simulink model "DIMR_ordinary"  (R2024b)
settings: Solver=daessc  StartTime=0.0  StopTime=20  RelTol=1e-3
values from neighbouring files (symbols this model uses):
  d_m0 = 0.12787808985686    (= 0.127878089857)    [DIMR_main.m]
  d_m_cmd = 0.12787808985686    (= 0.127878089857)    [DIMR_main.m]
  dis_cmd = 3    [DIMR_main.m]
  phi_cmd = 0*pi/180    (= 0)    [DIMR_main.m]
  theta_f0 = 0    [DIMR_main.m]
  theta_f_cmd = 0.037940459    [DIMR_main.m]
  theta_p0 = 0*pi/180    (= 0)    [DIMR_main.m]
  theta_p_cmd = -0.037940459    [DIMR_main.m]
undefined symbols (not defined in the file or in its folder): Ac, Dc, DiscIntNeverNeededParam, dspblkCoreblockFVToolHelper, g, g_ext, g_fork, g_lift, g_reac, g_spado, g_yaw, gcbh, K_fd, K_fp, K_md, K_mp, K_pd, K_pp, K_wd, K_wp, K_yd, K_yp, Kc, L_bx, L_by, L_bz, L_ex, L_ey, L_ez, L_fg, L_fh, L_fx, L_fy, L_fz, L_lx, L_ly, L_lz, L_mx, L_my, L_mz, L_wt, M_f, M_n11, M_n21, M_n22, M_n33, M_n44, Mc, N_f, N_w, omega_c, R_wi, R_wo, T_control, Torque_limit_f, Torque_limit_l, Torque_limit_w, W_w, X, Y ... (+1)
libraries: sm_lib x50, nesl_utility x12, simulink x9, slctrl_autotuning x1, slpidlib x1
(part 1 of 3)
settings Model: Creator=ITO  LastModifiedBy=Sergio Quintero
settings RTWCC: GPUComputeCapability=3.5

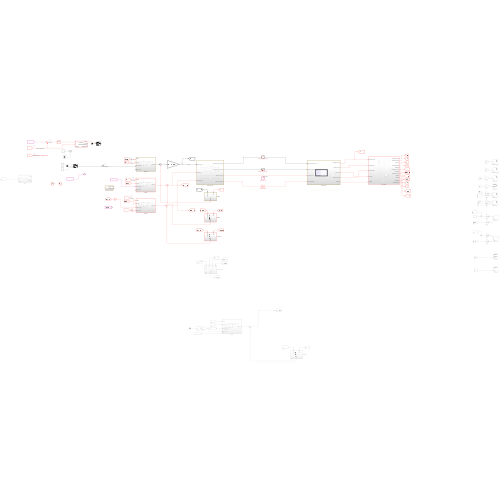
[thumbnail: Simulink's stored preview of the top-level diagram]
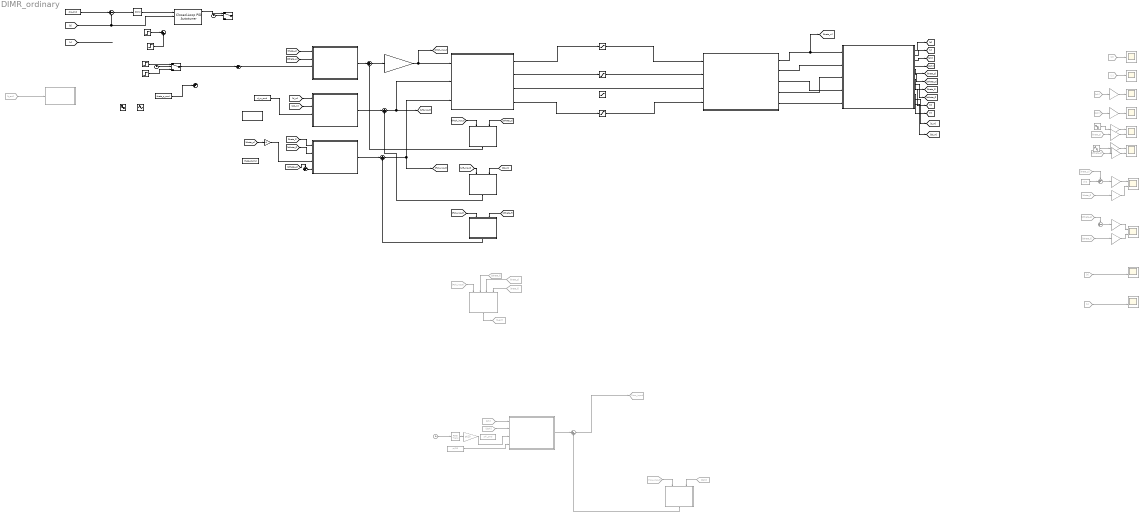
== system DIMR_ordinary ==
  Calc_states : Subsystem
  Clock : Clock  Commented=on
  Clock1 : Clock
  Clock2 : Clock
  Closed-Loop PID Autotuner : slctrl_autotuning/Closed-Loop PID Autotuner  PIDType=PD  PIDForm=Parallel  TimeDomain=discrete-time  DiscreteTs=T_control  TuningTs=0.2  UseTuningTs=off  IntegratorFormula=Forward Euler  FilterFormula=Forward Euler  ContinuousTs=0.02  Bandwidth=1  UseExternalWC=off  TargetPM=60  UseExternalPM=off  UseExternalAchievedPM=on  ExperimentMode=Superposition  PlantType=Stable  PlantSign=Positive  AmpSine=0.05  UseExternalAmpSine=off  UseExternalFRD=off  UseExternalU0=off  UseCompanion=off  NotDeployTuningModule=off  UsePLCCoder=off  OutputMode=control action + perturbation  BlockDataType=double  UseConnectedPID=on  blockpath=[]  tunedP=0  tunedI=0  tunedD=0  tunedN=100  tunedPM=0  EstimationWindowSize=3  UseExternalTuningParams=off  SingleMultiRateVariant=SingleSamplingRate  NumEstimationPeriods=4  NumSettlingPeriods=2  NumOfPRBSPeriod=1  PRBSSignalOrder=12  ExperimentModeVariant=VariantSuperimposed  OutputChoice=VariantCandD  ConvergenceCalcVariant=ConvSuperpositionPRBSVariant
      settings: LibrarySourceBlock=slctrlblks/Autotuning/Closed-Loop PID Autotuner
  Constant : Constant  Value=theta_p_cmd
  Constant1 : Constant  Commented=on  Value=phi_cmd
  Constant2 : Constant  Value=theta_f_cmd
  Constant3 : Constant  Commented=on  Value=pi/2
  Constant4 : Constant  Commented=on  Value=pi/20
  Constant5 : Constant  Value=d_m_cmd
  Constant6 : Constant  Value=dis_cmd
  Fork DOB : Subsystem
  Fork PD : Subsystem
  Fork position : Scope  Commented=on  NumInputPorts=2
  Fork velocity : Scope  Commented=on  NumInputPorts=2
  From1 : From  Commented=on  GotoTag=dphi
  From10 : From  Commented=on  GotoTag=Yaw_input
  From14 : From  Commented=on  GotoTag=d
  From15 : From  Commented=on  GotoTag=v
  From16 : From  Commented=on  GotoTag=phi
  From17 : From  Commented=on  GotoTag=dphi
  From18 : From  Commented=on  GotoTag=theta_p
  From19 : From  Commented=on  GotoTag=dtheta_p
  From20 : From  Commented=on  GotoTag=theta_f
  From21 : From  Commented=on  GotoTag=dtheta_f
  From22 : From  Commented=on  GotoTag=theta_p
  From23 : From  Commented=on  GotoTag=dtheta_p
  From24 : From  Commented=on  GotoTag=X
  From25 : From  Commented=on  GotoTag=Y
  From31 : From  Commented=on  GotoTag=dtheta_f
  From32 : From  Commented=on  GotoTag=Fork_input
  From33 : From  Commented=on  GotoTag=t_ext
  From34 : From  Commented=on  GotoTag=theta_p
  From35 : From  Commented=on  GotoTag=theta_f
  From5 : From  Commented=on  GotoTag=phi
  From6 : From  Commented=on  GotoTag=dphi
  Gain : Gain  Gain=-M_n11/(M_n21+M_n11)
  Gain{1..8,10..11} (10 alike) : Gain  Commented=on  Gain=180/pi
  Gain12 : Gain  Gain=-1
  Gain9 : Gain  Commented=on  Gain=pi/20
  Goto11 : Goto  Commented=on  GotoTag=Yaw_input
  Goto17 : Goto  Commented=on  GotoTag=t_ext
  Lift DOB : Subsystem
  Lift PD : Subsystem
  Lift movement profile : Subsystem
  PID Controller : slpidlib/PID Controller  Controller=PD  Form=Parallel  TimeDomain=Discrete-time  UseExternalTs=off  SampleTime=T_control  IntegratorMethod=Forward Euler  FilterMethod=Forward Euler  ControllerParametersSource=internal  P=K_wp  I=1  UseKiTs=off  D=K_wd  UseExternalDerivativeSource=off  N=100  UseFilter=off  TunerSelectOption=Transfer Function Based (PID Tuner App)  InitialConditionSource=internal  InitialConditionForIntegrator=0  InitialConditionForFilter=0  DifferentiatorICPrevScaledInput=0  ExternalReset=none  TrackingMode=off  Kt=1  LimitOutput=off  SatLimitsSource=internal  UpperSaturationLimit=inf  LowerSaturationLimit=-inf  LinearizeAsGain=on  AntiWindupMode=none  Kb=1  LimitIntegrator=off  UpperIntegratorSaturationLimit=inf  LowerIntegratorSaturationLimit=-inf  POutMin=[]  POutMax=[]  IOutMin=[]  IOutMax=[]  DOutMin=[]  DOutMax=[]  NOutMin=[]  NOutMax=[]  SumOutMin=[]  SumOutMax=[]  SaturationOutMin=[]  SaturationOutMax=[]  PParamMin=[]  PParamMax=[]  IParamMin=[]  IParamMax=[]  DParamMin=[]  DParamMax=[]  NParamMin=[]  NParamMax=[]  KbParamMin=[]  KbParamMax=[]  KtParamMin=[]  KtParamMax=[]  KbOutMin=[]  KbOutMax=[]  KtOutMin=[]  KtOutMax=[]  IntegratorOutMin=[]  IntegratorOutMax=[]  FilterOutMin=[]  FilterOutMax=[]  SumI1OutMin=[]  SumI1OutMax=[]  SumI2OutMin=[]  SumI2OutMax=[]  SumI3OutMin=[]  SumI3OutMax=[]  SumI4OutMin=[]  SumI4OutMax=[]  SumDOutMin=[]  SumDOutMax=[]  DifferentiatorOutMin=[]  DifferentiatorOutMax=[]  FilterDiffOutCoefMin=[]  FilterDiffOutCoefMax=[]  ReciprocalOutMin=[]  ReciprocalOutMax=[]  SumDenOutMin=[]  SumDenOutMax=[]  SumNumOutMin=[]  SumNumOutMax=[]  DivideOutMin=[]  DivideOutMax=[]  UdiffTsProdOutMin=[]  UdiffTsProdOutMax=[]  NTsProdOutMin=[]  NTsProdOutMax=[]  UintegralTsProdOutMin=[]  UintegralTsProdOutMax=[]  UngainTsProdOutMin=[]  UngainTsProdOutMax=[]  ClampingZeroOutDataTypeStr=Inherit: Inherit via back propagation  ClampingZeroOutMin=[]  ClampingZeroOutMax=[]  FilterDenConstantOutDataTypeStr=Inherit: Inherit via back propagation  FilterDenConstantOutMin=[]  FilterDenConstantOutMax=[]  PCopyOutDataTypeStr=Inherit: Inherit via back propagation  PCopyOutMin=[]  PCopyOutMax=[]  NCopyOutDataTypeStr=Inherit: Inherit via back propagation  NCopyOutMin=[]  NCopyOutMax=[]  IntegratorContinuousStateAttributes=''  IntegratorStateMustResolveToSignalObject=off  IntegratorRTWStateStorageClass=Auto  FilterContinuousStateAttributes=''  FilterStateMustResolveToSignalObject=off  FilterRTWStateStorageClass=Auto  ParallelPVariant=InternalParameters  IdealPVariant=Disabled  IVariant=Disabled  DVariant=InternalParameters  IntegratorVariant=Disabled  SatVariant=Disabled  AWVariant=Disabled  PCopyVariant=Disabled  TRVariant=Disabled  FdbkBlocksVariant=Forward  IdealPFdbkVariant=Disabled  SatFdbkVariant=Disabled  DerivativeFilterVariant=Differentiator  NVariant=Passthrough  NCopyVariant=Disabled_SignalSpec  FilterICVariant=InternalICsDifferentiator  IntegratorICVariant=Disabled  ExternalResetVariant=Disabled  TRSumVariant=Passthrough  SumFdbkVariant=Disabled  SumVariant=Sum_PD  TsampFilterVariant=InternalTs  TsampNgainVariant=Passthrough  TsampIntegralVariant=Disabled_SignalSpec  ExternalSaturationOutDataTypeStr=Inherit: Same as second input  DerivativeSourceVariant=ErrorSignal  PreIntVariant=InternalPreInt
  Pitch PD : Subsystem
  Pitch position : Scope  Commented=on  NumInputPorts=2
  Pitch velocity : Scope  Commented=on  NumInputPorts=2
  Plant model : Subsystem
  RCC : Subsystem  Commented=on
  Rate Transition : RateTransition  Commented=on  OutPortSampleTime=T_control
  Reaction DOB : Subsystem  Commented=on
  SPADO : Subsystem
  Sine Wave : Sin  Amplitude=10*pi/180  SampleTime=T_control
  Sine Wave1 : Sin  Amplitude=10*pi/180  Phase=pi/2  SampleTime=T_control
  Sine Wave2 : Sin  Commented=on  Amplitude=10*pi/180  SampleTime=T_control
  Sine Wave3 : Sin  Commented=on  Amplitude=10*pi/180  Phase=pi/2  SampleTime=T_control
  Step : Step  Time=10  SampleTime=0
  Step1 : Step  Time=20  After=-1  SampleTime=0
  Step2 : Step  Time=0  After=theta_p_cmd*3/2  SampleTime=0
  Step3 : Step  Time=0  After=theta_p_cmd/2  SampleTime=0
  Sum{,2,7,10} (4 alike) : Sum  Inputs=|++
  Sum1 : Sum  Commented=on  Inputs=|++
  Sum3 : Sum  Inputs=++|
  Sum4 : Sum  Inputs=-+|
  Sum5 : Sum  Commented=on  Inputs=-+|
  Sum6 : Sum  Commented=on  Inputs=-+|
  Sum8 : Sum  Inputs=++|
  Sum9 : Sum  Inputs=|+-
  Switch : Switch  Criteria=u2 > Threshold  Threshold=5  SaturateOnIntegerOverflow=off  InputSameDT=off
  Switch1 : Switch  Criteria=u2 > Threshold  Threshold=5  SaturateOnIntegerOverflow=off  InputSameDT=off
  Transform_input : Subsystem
  Translational position : Scope  Commented=on
  Translational velocity : Scope  Commented=on
  X position : Scope  Commented=on  NumInputPorts=2
  Y position : Scope  Commented=on  NumInputPorts=2
  Yaw DOB : Subsystem  Commented=on
  Yaw PD : Subsystem  Commented=on
  Yaw Position : Scope  Commented=on
  Yaw rate : Scope  Commented=on
  torque_limit_fork : Saturate  UpperLimit=Torque_limit_f  LowerLimit=-Torque_limit_f
  torque_limit_left_wheel : Saturate  UpperLimit=Torque_limit_w  LowerLimit=-Torque_limit_w
  torque_limit_lift : Saturate  UpperLimit=Torque_limit_l  LowerLimit=-Torque_limit_l
  torque_limit_right_wheel : Saturate  UpperLimit=Torque_limit_w  LowerLimit=-Torque_limit_w
  wires:
  Plant model/4(Pitch_Euler_Angle) -> Calc_states/3(Pitch euler angle)
  Plant model/3(Fork_Angle) -> Calc_states/4(Fork angle)
  torque_limit_left_wheel/1 -> Plant model/2(Left_wheel_motor_torque)
  Plant model/1(Right_Wheel_Angle) -> [theta_w], Calc_states/1(Right wheel angle)
  Transform_input/4(Fork_motor_torque_ref) -> torque_limit_fork/1
  torque_limit_right_wheel/1 -> Plant model/1(Right_wheel_motor_torque)
  torque_limit_fork/1 -> Plant model/4(Fork_motor_torque)
  Transform_input/1(Right_wheel_motor_torque_ref) -> torque_limit_right_wheel/1
  Transform_input/2(Left_wheel_motor_torque_ref) -> torque_limit_left_wheel/1
  Plant model/2(Left_Wheel_Angle) -> Calc_states/2(Left wheel angle)
  Gain/1 -> [Pitch_input], Transform_input/1(Pitch_torque_ref)  "Tp_ref"
  Pitch PD/1(Torque_ref) -> Sum/1
  Sum/1 -> Gain/1
  Yaw PD/1(Torque_ref) -> Sum1/1
  Sum1/1 -> Goto11/1
  Yaw DOB/1(Est_dis) -> Sum1/2
  Fork PD/1(Torque_ref) -> Sum2/1
  Sum2/1 -> [Fork_input], Transform_input/3(Fork_torque_ref)
  Calc_states/1(Translational position) -> [d]
  Calc_states/2(Translational velocity) -> [v]
  Calc_states/3(Yaw angle) -> [phi]
  Calc_states/4(Yaw angular velocity) -> [dphi]
  Calc_states/5(Pitch angle) -> [theta_p]
  Calc_states/6(Pitch angular velocity) -> [dtheta_p]
  Calc_states/7(Fork position) -> [theta_f]
  Calc_states/8(Fork angular velocity) -> [dtheta_f]
  Calc_states/9(X position) -> [X]
  Calc_states/10(Y position) -> [Y]
  [dtheta_p] -> SPADO/2(Velocity)
  From1/1 -> Yaw DOB/2(Velocity)
  [dtheta_f] -> Fork DOB/2(Velocity)
  [dtheta_p] -> Pitch PD/2(Velocity)  "Pitch ang vel"
  [theta_p] -> Pitch PD/1(Position)  "Pitch angle"
  From5/1 -> Yaw PD/1(Position)
  From6/1 -> Yaw PD/2(Velocity)
  [theta_f] -> Fork PD/1(Position)  "Fork angle"
  [dtheta_f] -> Fork PD/2(Velocity)
  [Pitch_input] -> SPADO/1(Input Torque)
  From10/1 -> Yaw DOB/1(Input Torque)
  [Fork_input] -> Fork DOB/1(Input Torque)
  Sum4/1 -> Fork PD/4(Velocity_cmd)
  [theta_p] -> Gain12/1
  [dtheta_p] -> Sum4/1
  From14/1 -> Translational position/1  "res"
  From15/1 -> Translational velocity/1  "res"
  From16/1 -> Gain1/1
  From17/1 -> Gain2/1
  From18/1 -> Gain3/1
  From19/1 -> Gain4/1
  From20/1 -> Gain6/1
  From21/1 -> Gain8/1
  Sum5/1 -> Gain5/1
  Sum6/1 -> Gain7/1
  From22/1 -> Sum5/1
  Constant3/1 -> Sum5/2
  From23/1 -> Sum6/1
  Gain1/1 -> Yaw Position/1  "res"
  Gain2/1 -> Yaw rate/1  "res"
  Gain3/1 -> Pitch position/2  "res"
  Gain4/1 -> Pitch velocity/2  "res"
  Gain5/1 -> Fork position/1  "cmd"
  Gain6/1 -> Fork position/2  "res"
  Gain7/1 -> Fork velocity/1  "cmd"
  Gain8/1 -> Fork velocity/2  "res"
  Fork DOB/1(Est_dis) -> Sum2/2
  From24/1 -> X position/2  "res"
  From25/1 -> Y position/2  "res"
  Clock/1 -> Rate Transition/1
  Gain9/1 -> Yaw PD/3(Position_cmd)
  Rate Transition/1 -> Gain9/1
  Constant4/1 -> Yaw PD/4(Velocity_cmd)
  Gain10/1 -> Pitch position/1  "res"
  Sine Wave2/1 -> Gain10/1
  Gain11/1 -> Pitch velocity/1  "res"
  Sine Wave3/1 -> Gain11/1
  Lift PD/1(Torque_ref) -> Sum7/1
  Lift DOB/1(Est_dis) -> Sum7/2
  Sum7/1 -> [Lift_input], Transform_input/2(Lift_force_ref)
  [Lift_input] -> Lift DOB/1(Input Torque)
  Plant model/5(Lift_height) -> Calc_states/5(Lift height)
  Calc_states/11(Lift position) -> [d_m]
  Calc_states/12(Lift linear velocity) -> [dd_m]
  [dd_m] -> Lift DOB/2(Velocity)
  [d_m] -> Lift PD/1(Position)  "Lift_height"
  [dd_m] -> Lift PD/2(Velocity)
  Transform_input/3(Lift_motor_torque_ref) -> Plant model/3(Lift_motor_torque)  "Control height"
  [d] -> Closed-Loop PID Autotuner/2, Sum9/2  "Horizontal displacement"
  From31/1 -> Reaction DOB/2(Velocity)
  From32/1 -> Reaction DOB/1(Input Torque)
  Reaction DOB/1(Est_dis) -> Goto17/1
  From33/1 -> RCC/1(t_ext)
  From34/1 -> Reaction DOB/3(Theta_p)
  From35/1 -> Reaction DOB/4(Theta_f)
  Sum9/1 -> PID Controller/1  "Pos_error"
  PID Controller/1 -> Closed-Loop PID Autotuner/1
  Step/1 -> Sum10/1
  Step1/1 -> Sum10/2
  Constant6/1 -> Sum9/1
  Constant/1 -> Sum8/2
  Gain12/1 -> Fork PD/3(Position_cmd)
  Clock1/1 -> Switch/2
  Clock2/1 -> Switch1/2
  SPADO/1(Est_dis) -> Sum/2
  Sum3/1 -> Pitch PD/3(Position_cmd)  "Total_pitch"
  Step2/1 -> Switch/1
  Step3/1 -> Switch/3
  [v] -> ?  "Horizontal velocity"
  Switch/1 -> Sum3/2
  Constant5/1 -> Lift PD/3(Position_cmd)
  Closed-Loop PID Autotuner/1 -> Switch1/1

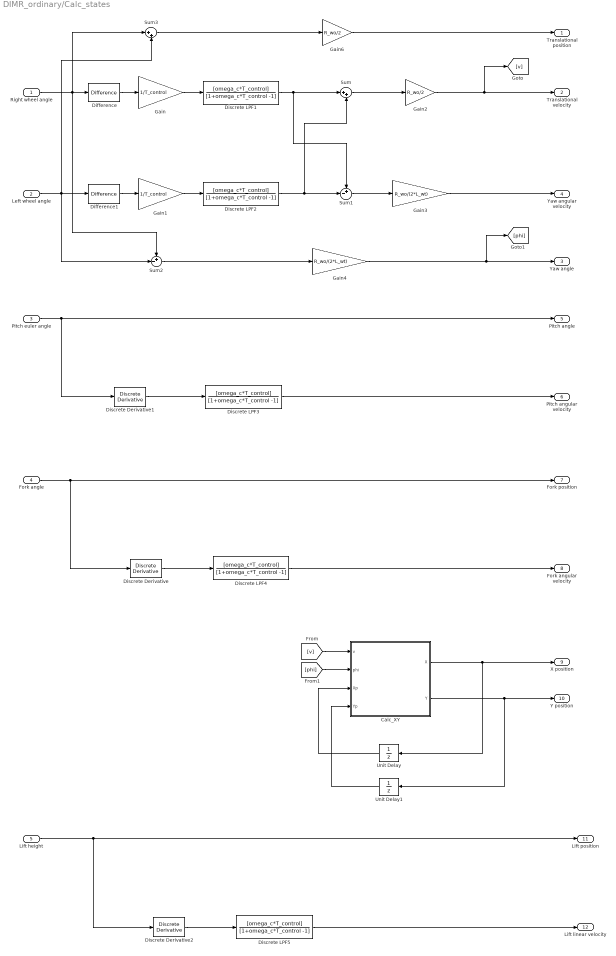
== system DIMR_ordinary/Calc_states ==
  Right wheel angle : Inport
  Left wheel angle : Inport  Port=2
  Pitch euler angle : Inport  Port=3
  Fork angle : Inport  Port=4
  Lift height : Inport  Port=5
  Calc_XY : MATLAB Function  TreatAsAtomicUnit=on
  Difference : simulink/Discrete/Difference  ICPrevInput=0.0  OutMin=[]  OutMax=[]  OutDataType=fixdt(1, 16)  OutScaling=2^-10  DoSatur=off
  Difference1 : simulink/Discrete/Difference  ICPrevInput=0.0  OutMin=[]  OutMax=[]  OutDataType=fixdt(1, 16)  OutScaling=2^-10  DoSatur=off
  Discrete Derivative : simulink/Discrete/Discrete Derivative  gainval=1.0  ICPrevScaledInput=theta_f0/T_control  OutMin=[]  OutMax=[]  OutDataType=fixdt(1, 16)  OutScaling=2^-10  DoSatur=off
  Discrete Derivative1 : simulink/Discrete/Discrete Derivative  gainval=1.0  ICPrevScaledInput=theta_p0/T_control  OutMin=[]  OutMax=[]  OutDataType=fixdt(1, 16)  OutScaling=2^-10  DoSatur=off
  Discrete Derivative2 : simulink/Discrete/Discrete Derivative  gainval=1.0  ICPrevScaledInput=d_m0/T_control  OutMin=[]  OutMax=[]  OutDataType=fixdt(1, 16)  OutScaling=2^-10  DoSatur=off
  Discrete LPF1 : DiscreteFilter  LoadFcn=dspblkCoreblockFVToolHelper(gcbh,'load');  Numerator=[omega_c*T_control]  Denominator=[1+omega_c*T_control -1]
      settings: CopyFcn=dspblkCoreblockFVToolHelper(gcbh,'copy');  DeleteFcn=dspblkCoreblockFVToolHelper(gcbh,'close');  ModelCloseFcn=dspblkCoreblockFVToolHelper(gcbh,'close');  PreSaveFcn=dspblkCoreblockFVToolHelper(gcbh,'presave');  PostSaveFcn=dspblkCoreblockFVToolHelper(gcbh,'postsave');  CloseFcn=dspblkCoreblockFVToolHelper(gcbh,'close');
  Discrete LPF2 : DiscreteFilter  Numerator=[omega_c*T_control]  Denominator=[1+omega_c*T_control -1]
  Discrete LPF3 : DiscreteFilter  Numerator=[omega_c*T_control]  Denominator=[1+omega_c*T_control -1]
  Discrete LPF4 : DiscreteFilter  Numerator=[omega_c*T_control]  Denominator=[1+omega_c*T_control -1]
  Discrete LPF5 : DiscreteFilter  LoadFcn=dspblkCoreblockFVToolHelper(gcbh,'load');  Numerator=[omega_c*T_control]  Denominator=[1+omega_c*T_control -1]
      settings: CopyFcn=dspblkCoreblockFVToolHelper(gcbh,'copy');  DeleteFcn=dspblkCoreblockFVToolHelper(gcbh,'close');  ModelCloseFcn=dspblkCoreblockFVToolHelper(gcbh,'close');  PreSaveFcn=dspblkCoreblockFVToolHelper(gcbh,'presave');  PostSaveFcn=dspblkCoreblockFVToolHelper(gcbh,'postsave');  CloseFcn=dspblkCoreblockFVToolHelper(gcbh,'close');
  Gain : Gain  Gain=1/T_control
  Gain1 : Gain  Gain=1/T_control
  Gain2 : Gain  Gain=R_wo/2
  Gain3 : Gain  Gain=R_wo/(2*L_wt)
  Gain4 : Gain  Gain=R_wo/(2*L_wt)
  Gain6 : Gain  Gain=R_wo/2
  Sum : Sum  Inputs=|++
  Sum1 : Sum  Inputs=+-|
  Sum2 : Sum  Inputs=+-|
  Sum3 : Sum  Inputs=|++
  Unit Delay : UnitDelay  SampleTime=T_control  HasFrameUpgradeWarning=on
  Unit Delay1 : UnitDelay  SampleTime=T_control  HasFrameUpgradeWarning=on
  Translational position : Outport
  Translational velocity : Outport  Port=2
  Yaw angle : Outport  Port=3
  Yaw angular velocity : Outport  Port=4
  Pitch angle : Outport  Port=5
  Pitch angular velocity : Outport  Port=6
  Fork position : Outport  Port=7
  Fork angular velocity : Outport  Port=8
  X position : Outport  Port=9
  Y position : Outport  Port=10
  Lift position : Outport  Port=11
  Lift linear velocity : Outport  Port=12
  wires:
  Right wheel angle/1 -> Sum3/1, Sum2/1, Difference/1
  Difference/1 -> Gain/1
  Gain/1 -> Discrete LPF1/1
  Difference1/1 -> Gain1/1
  Gain1/1 -> Discrete LPF2/1
  Left wheel angle/1 -> Sum3/2, Sum2/2, Difference1/1
  Discrete LPF1/1 -> Sum/1, Sum1/1
  Discrete LPF2/1 -> Sum1/2, Sum/2
  Sum/1 -> Gain2/1
  Gain2/1 -> Translational velocity/1, [v]
  Sum1/1 -> Gain3/1
  Gain3/1 -> Yaw angular velocity/1
  Sum2/1 -> Gain4/1
  Gain4/1 -> [phi], Yaw angle/1
  Discrete Derivative1/1 -> Discrete LPF3/1
  Discrete LPF3/1 -> Pitch angular velocity/1
  Pitch euler angle/1 -> Discrete Derivative1/1, Pitch angle/1
  Sum3/1 -> Gain6/1
  Gain6/1 -> Translational position/1
  Discrete Derivative/1 -> Discrete LPF4/1
  Fork angle/1 -> Discrete Derivative/1, Fork position/1
  Discrete LPF4/1 -> Fork angular velocity/1
  [v] -> Calc_XY/1(v)
  [phi] -> Calc_XY/2(phi)
  Calc_XY/1(X) -> Unit Delay/1, X position/1
  Calc_XY/2(Y) -> Unit Delay1/1, Y position/1
  Unit Delay/1 -> Calc_XY/3(Xp)
  Unit Delay1/1 -> Calc_XY/4(Yp)
  Discrete LPF5/1 -> Lift linear velocity/1
  Lift height/1 -> Lift position/1, Discrete Derivative2/1
  Discrete Derivative2/1 -> Discrete LPF5/1

== system DIMR_ordinary/Fork DOB ==
  Input Torque : Inport
  Velocity : Inport  Port=2
  Discrete LPF1 : DiscreteFilter  Numerator=[g_fork*T_control]  Denominator=[1+g_fork*T_control -1]
  Gain8 : Gain  Gain=g_fork*M_n44
  Scope5 : Scope
  Sum5 : Sum  Inputs=+|+
  Sum6 : Sum  Inputs=|+-
  Est_dis : Outport
  wires:
  Velocity/1 -> Gain8/1
  Discrete LPF1/1 -> Sum6/1
  Gain8/1 -> Sum6/2, Sum5/2
  Input Torque/1 -> Sum5/1
  Sum6/1 -> Est_dis/1, Scope5/1
  Sum5/1 -> Discrete LPF1/1

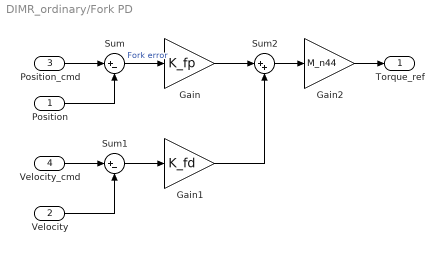
== system DIMR_ordinary/Fork PD ==
  Position : Inport
  Velocity : Inport  Port=2
  Position_cmd : Inport  Port=3
  Velocity_cmd : Inport  Port=4
  Gain : Gain  Gain=K_fp
  Gain1 : Gain  Gain=K_fd
  Gain2 : Gain  Gain=M_n44
  Sum : Sum  Inputs=|+-
  Sum1 : Sum  Inputs=|+-
  Sum2 : Sum  Inputs=|++
  Torque_ref : Outport
  wires:
  Sum/1 -> Gain/1  "Fork error"
  Position/1 -> Sum/2
  Position_cmd/1 -> Sum/1
  Sum1/1 -> Gain1/1
  Velocity/1 -> Sum1/2
  Gain/1 -> Sum2/1
  Gain1/1 -> Sum2/2
  Sum2/1 -> Gain2/1
  Gain2/1 -> Torque_ref/1
  Velocity_cmd/1 -> Sum1/1

== system DIMR_ordinary/Lift DOB ==
  Input Torque : Inport
  Velocity : Inport  Port=2
  Discrete LPF1 : DiscreteFilter  LoadFcn=dspblkCoreblockFVToolHelper(gcbh,'load');  Numerator=[g_lift*T_control]  Denominator=[1+g_lift*T_control -1]
      settings: CopyFcn=dspblkCoreblockFVToolHelper(gcbh,'copy');  DeleteFcn=dspblkCoreblockFVToolHelper(gcbh,'close');  ModelCloseFcn=dspblkCoreblockFVToolHelper(gcbh,'close');  PreSaveFcn=dspblkCoreblockFVToolHelper(gcbh,'presave');  PostSaveFcn=dspblkCoreblockFVToolHelper(gcbh,'postsave');  CloseFcn=dspblkCoreblockFVToolHelper(gcbh,'close');
  Gain8 : Gain  Gain=g_lift*M_n33
  Scope5 : Scope
  Sum5 : Sum  Inputs=+|+
  Sum6 : Sum  Inputs=|+-
  Est_dis : Outport
  wires:
  Sum5/1 -> Discrete LPF1/1
  Sum6/1 -> Scope5/1, Est_dis/1
  Input Torque/1 -> Sum5/1
  Gain8/1 -> Sum5/2, Sum6/2
  Discrete LPF1/1 -> Sum6/1
  Velocity/1 -> Gain8/1

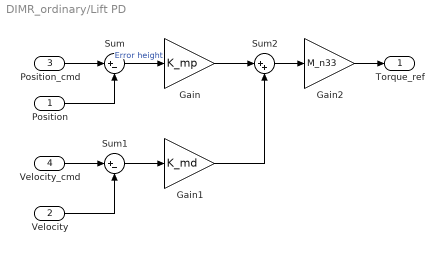
== system DIMR_ordinary/Lift PD ==
  Position : Inport
  Velocity : Inport  Port=2
  Position_cmd : Inport  Port=3
  Velocity_cmd : Inport  Port=4
  Gain : Gain  Gain=K_mp
  Gain1 : Gain  Gain=K_md
  Gain2 : Gain  Gain=M_n33
  Sum : Sum  Inputs=|+-
  Sum1 : Sum  Inputs=|+-
  Sum2 : Sum  Inputs=|++
  Torque_ref : Outport
  wires:
  Velocity_cmd/1 -> Sum1/1
  Gain2/1 -> Torque_ref/1
  Sum2/1 -> Gain2/1
  Gain1/1 -> Sum2/2
  Gain/1 -> Sum2/1
  Velocity/1 -> Sum1/2
  Sum1/1 -> Gain1/1
  Position_cmd/1 -> Sum/1
  Position/1 -> Sum/2
  Sum/1 -> Gain/1  "Error height"

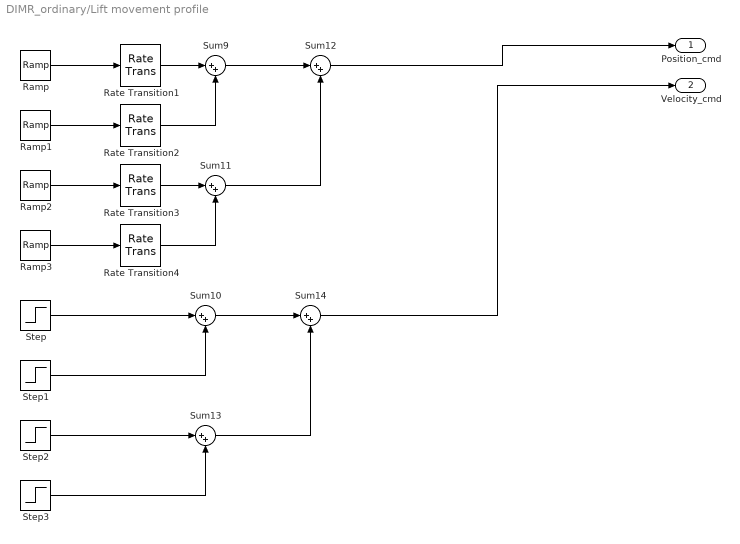
== system DIMR_ordinary/Lift movement profile ==
  Ramp : simulink/Sources/Ramp  slope=-0.2/4  start=6  InitialOutput=d_m_cmd
  Ramp1 : simulink/Sources/Ramp  slope=0.2/4  start=9  InitialOutput=0
  Ramp2 : simulink/Sources/Ramp  slope=0.2/4  start=14  InitialOutput=0
  Ramp3 : simulink/Sources/Ramp  slope=-0.2/4  start=17  InitialOutput=0
  Rate Transition{1..4} (4 alike) : RateTransition  OutPortSampleTime=T_control
  Step : Step  Time=6  After=-0.2/4  SampleTime=T_control
  Step1 : Step  Time=9  After=0.2/4  SampleTime=T_control
  Step2 : Step  Time=14  After=0.2/4  SampleTime=T_control
  Step3 : Step  Time=17  After=-0.2/4  SampleTime=T_control
  Sum{9..14} (6 alike) : Sum  Inputs=|++
  Position_cmd : Outport
  Velocity_cmd : Outport  Port=2
  wires:
  Rate Transition4/1 -> Sum11/2
  Sum9/1 -> Sum12/1
  Ramp1/1 -> Rate Transition2/1
  Sum11/1 -> Sum12/2
  Sum13/1 -> Sum14/2
  Ramp/1 -> Rate Transition1/1
  Step3/1 -> Sum13/2
  Step2/1 -> Sum13/1
  Rate Transition1/1 -> Sum9/1
  Step/1 -> Sum10/1
  Step1/1 -> Sum10/2
  Rate Transition3/1 -> Sum11/1
  Rate Transition2/1 -> Sum9/2
  Sum10/1 -> Sum14/1
  Ramp2/1 -> Rate Transition3/1
  Ramp3/1 -> Rate Transition4/1
  Sum12/1 -> Position_cmd/1
  Sum14/1 -> Velocity_cmd/1

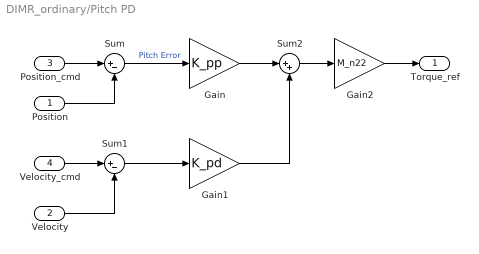
== system DIMR_ordinary/Pitch PD ==
  Position : Inport
  Velocity : Inport  Port=2
  Position_cmd : Inport  Port=3
  Velocity_cmd : Inport  Port=4
  Gain : Gain  Gain=K_pp
  Gain1 : Gain  Gain=K_pd
  Gain2 : Gain  Gain=M_n22
  Sum : Sum  Inputs=|+-
  Sum1 : Sum  Inputs=|+-
  Sum2 : Sum  Inputs=|++
  Torque_ref : Outport
  wires:
  Sum/1 -> Gain/1  "Pitch Error"
  Position/1 -> Sum/2
  Position_cmd/1 -> Sum/1
  Sum1/1 -> Gain1/1
  Velocity_cmd/1 -> Sum1/1
  Velocity/1 -> Sum1/2
  Gain/1 -> Sum2/1
  Gain1/1 -> Sum2/2
  Sum2/1 -> Gain2/1
  Gain2/1 -> Torque_ref/1

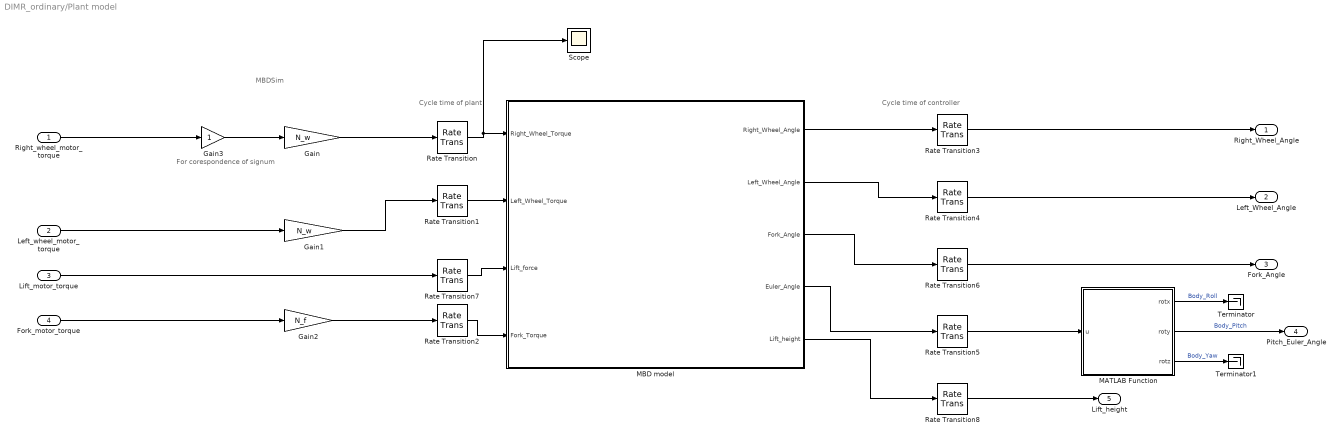
== system DIMR_ordinary/Plant model ==
  note: Cycle time of controller
  note: MBDSim
  note: For corespondence of signum
  note: Cycle time of plant
  Right_wheel_motor_torque : Inport
  Left_wheel_motor_torque : Inport  Port=2
  Lift_motor_torque : Inport  Port=3
  Fork_motor_torque : Inport  Port=4
  Gain : Gain  Gain=N_w
  Gain1 : Gain  Gain=N_w
  Gain2 : Gain  Gain=N_f
  Gain3 : Gain
  MATLAB Function : MATLAB Function  TreatAsAtomicUnit=on
  MBD model : Subsystem
  Rate Transition{,1..8} (9 alike) : RateTransition  OutPortSampleTime=T_control
  Scope : Scope
  Terminator : Terminator
  Terminator1 : Terminator
  Right_Wheel_Angle : Outport
  Left_Wheel_Angle : Outport  Port=2
  Fork_Angle : Outport  Port=3
  Pitch_Euler_Angle : Outport  Port=4
  Lift_height : Outport  Port=5
  wires:
  Rate Transition/1 -> Scope/1, MBD model/1(Right_Wheel_Torque)
  MBD model/3(Fork_Angle) -> Rate Transition6/1
  Gain3/1 -> Gain/1
  MBD model/1(Right_Wheel_Angle) -> Rate Transition3/1
  Rate Transition1/1 -> MBD model/2(Left_Wheel_Torque)
  Fork_motor_torque/1 -> Gain2/1
  MBD model/2(Left_Wheel_Angle) -> Rate Transition4/1
  Gain/1 -> Rate Transition/1
  MBD model/4(Euler_Angle) -> Rate Transition5/1
  Rate Transition2/1 -> MBD model/4(Fork_Torque)
  Gain2/1 -> Rate Transition2/1
  Gain1/1 -> Rate Transition1/1
  Left_wheel_motor_torque/1 -> Gain1/1
  Right_wheel_motor_torque/1 -> Gain3/1
  Rate Transition4/1 -> Left_Wheel_Angle/1
  Rate Transition3/1 -> Right_Wheel_Angle/1
  Rate Transition6/1 -> Fork_Angle/1
  MATLAB Function/1(rotx) -> Terminator/1  "Body_Roll"
  MATLAB Function/3(rotz) -> Terminator1/1  "Body_Yaw"
  Rate Transition5/1 -> MATLAB Function/1(u)
  MATLAB Function/2(roty) -> Pitch_Euler_Angle/1  "Body_Pitch"
  Lift_motor_torque/1 -> Rate Transition7/1
  Rate Transition8/1 -> Lift_height/1
  MBD model/5(Lift_height) -> Rate Transition8/1
  Rate Transition7/1 -> MBD model/3(Lift_force)

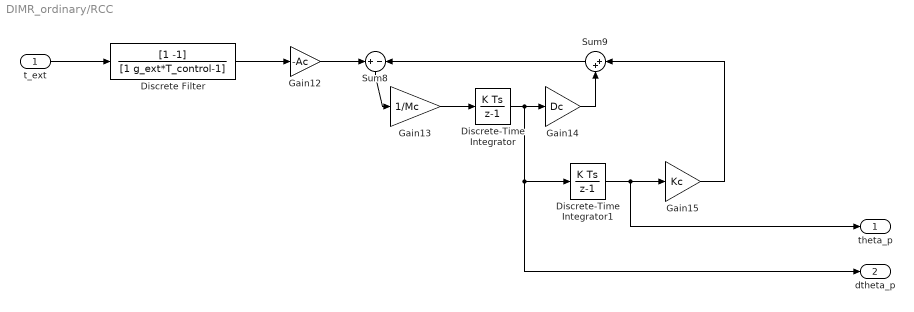
== system DIMR_ordinary/RCC ==
  t_ext : Inport
  Discrete Filter : DiscreteFilter  LoadFcn=dspblkCoreblockFVToolHelper(gcbh,'load');  Numerator=[1 -1]  Denominator=[1 g_ext*T_control-1]
      settings: CopyFcn=dspblkCoreblockFVToolHelper(gcbh,'copy');  DeleteFcn=dspblkCoreblockFVToolHelper(gcbh,'close');  ModelCloseFcn=dspblkCoreblockFVToolHelper(gcbh,'close');  PreSaveFcn=dspblkCoreblockFVToolHelper(gcbh,'presave');  PostSaveFcn=dspblkCoreblockFVToolHelper(gcbh,'postsave');  CloseFcn=dspblkCoreblockFVToolHelper(gcbh,'close');
  Discrete-Time Integrator : DiscreteIntegrator  SampleTime=T_control  ICPrevOutput=DiscIntNeverNeededParam  ICPrevScaledInput=DiscIntNeverNeededParam
  Discrete-Time Integrator1 : DiscreteIntegrator  SampleTime=T_control  ICPrevOutput=DiscIntNeverNeededParam  ICPrevScaledInput=DiscIntNeverNeededParam
  Gain12 : Gain  Gain=-Ac
  Gain13 : Gain  Gain=1/Mc
  Gain14 : Gain  Gain=Dc
  Gain15 : Gain  Gain=Kc
  Sum8 : Sum  Inputs=+-
  Sum9 : Sum  Inputs=|++
  theta_p : Outport
  dtheta_p : Outport  Port=2
  wires:
  Gain14/1 -> Sum9/2
  Discrete-Time Integrator1/1 -> theta_p/1, Gain15/1
  Gain13/1 -> Discrete-Time Integrator/1
  Sum8/1 -> Gain13/1
  Gain15/1 -> Sum9/1
  Sum9/1 -> Sum8/2
  Discrete-Time Integrator/1 -> Discrete-Time Integrator1/1, dtheta_p/1, Gain14/1
  Gain12/1 -> Sum8/1
  t_ext/1 -> Discrete Filter/1
  Discrete Filter/1 -> Gain12/1

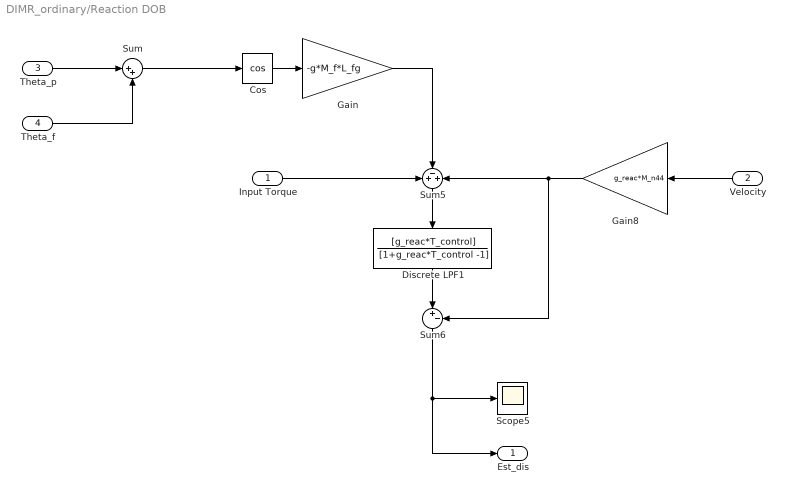
== system DIMR_ordinary/Reaction DOB ==
  Input Torque : Inport
  Velocity : Inport  Port=2
  Theta_p : Inport  Port=3
  Theta_f : Inport  Port=4
  Cos : Trigonometry  Operator=cos
  Discrete LPF1 : DiscreteFilter  LoadFcn=dspblkCoreblockFVToolHelper(gcbh,'load');  Numerator=[g_reac*T_control]  Denominator=[1+g_reac*T_control -1]
      settings: CopyFcn=dspblkCoreblockFVToolHelper(gcbh,'copy');  DeleteFcn=dspblkCoreblockFVToolHelper(gcbh,'close');  ModelCloseFcn=dspblkCoreblockFVToolHelper(gcbh,'close');  PreSaveFcn=dspblkCoreblockFVToolHelper(gcbh,'presave');  PostSaveFcn=dspblkCoreblockFVToolHelper(gcbh,'postsave');  CloseFcn=dspblkCoreblockFVToolHelper(gcbh,'close');
  Gain : Gain  Gain=-g*M_f*L_fg
  Gain8 : Gain  Gain=g_reac*M_n44
  Scope5 : Scope
  Sum : Sum  Inputs=|++
  Sum5 : Sum  Inputs=+-+
  Sum6 : Sum  Inputs=|+-
  Est_dis : Outport
  wires:
  Sum5/1 -> Discrete LPF1/1
  Sum6/1 -> Scope5/1, Est_dis/1
  Input Torque/1 -> Sum5/1
  Gain8/1 -> Sum5/3, Sum6/2
  Discrete LPF1/1 -> Sum6/1
  Velocity/1 -> Gain8/1
  Cos/1 -> Gain/1
  Gain/1 -> Sum5/2
  Theta_p/1 -> Sum/1
  Theta_f/1 -> Sum/2
  Sum/1 -> Cos/1

== system DIMR_ordinary/SPADO ==
  Input Torque : Inport
  Velocity : Inport  Port=2
  Discrete LPF1 : DiscreteFilter  Numerator=[g_spado*T_control]  Denominator=[1+g_spado*T_control -1]
  Gain1 : Gain  Gain=(M_n21+M_n11)/M_n11
  Gain8 : Gain  Gain=g_spado*M_n22
  Scope5 : Scope
  Sum5 : Sum  Inputs=-|+
  Sum6 : Sum  Inputs=|+-
  Est_dis : Outport
  wires:
  Velocity/1 -> Gain8/1
  Discrete LPF1/1 -> Sum6/1
  Gain8/1 -> Sum6/2, Sum5/2
  Sum6/1 -> Est_dis/1, Scope5/1
  Sum5/1 -> Discrete LPF1/1
  Gain1/1 -> Sum5/1
  Input Torque/1 -> Gain1/1

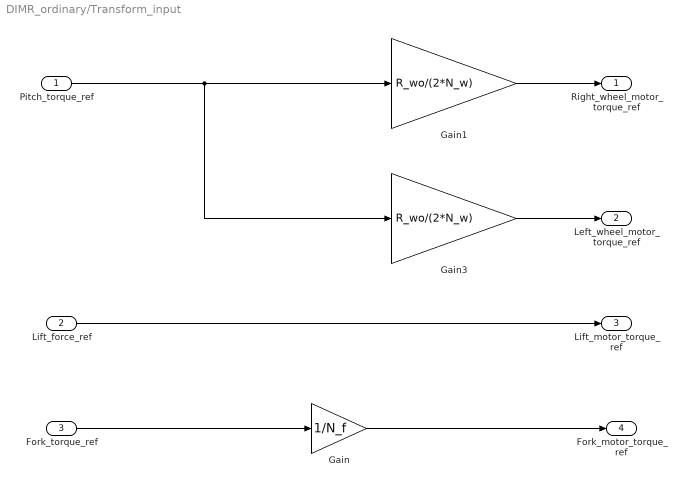
== system DIMR_ordinary/Transform_input ==
  Pitch_torque_ref : Inport
  Lift_force_ref : Inport  Port=2
  Fork_torque_ref : Inport  Port=3
  Gain : Gain  Gain=1/N_f
  Gain1 : Gain  Gain=R_wo/(2*N_w)
  Gain3 : Gain  Gain=R_wo/(2*N_w)
  Right_wheel_motor_torque_ref : Outport
  Left_wheel_motor_torque_ref : Outport  Port=2
  Lift_motor_torque_ref : Outport  Port=3
  Fork_motor_torque_ref : Outport  Port=4
  wires:
  Fork_torque_ref/1 -> Gain/1
  Gain/1 -> Fork_motor_torque_ref/1
  Gain1/1 -> Right_wheel_motor_torque_ref/1
  Pitch_torque_ref/1 -> Gain3/1, Gain1/1
  Gain3/1 -> Left_wheel_motor_torque_ref/1
  Lift_force_ref/1 -> Lift_motor_torque_ref/1

== system DIMR_ordinary/Yaw DOB ==
  Input Torque : Inport
  Velocity : Inport  Port=2
  Discrete LPF1 : DiscreteFilter  Numerator=[g_yaw*T_control]  Denominator=[1+g_yaw*T_control -1]
  Gain8 : Gain  Gain=g_yaw*M_n22
  Scope5 : Scope
  Sum5 : Sum  Inputs=+|+
  Sum6 : Sum  Inputs=|+-
  Est_dis : Outport
  wires:
  Velocity/1 -> Gain8/1
  Discrete LPF1/1 -> Sum6/1
  Gain8/1 -> Sum6/2, Sum5/2
  Input Torque/1 -> Sum5/1
  Sum6/1 -> Est_dis/1, Scope5/1
  Sum5/1 -> Discrete LPF1/1

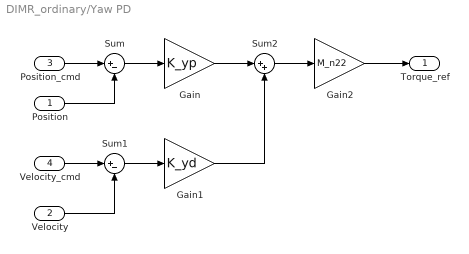
== system DIMR_ordinary/Yaw PD ==
  Position : Inport
  Velocity : Inport  Port=2
  Position_cmd : Inport  Port=3
  Velocity_cmd : Inport  Port=4
  Gain : Gain  Gain=K_yp
  Gain1 : Gain  Gain=K_yd
  Gain2 : Gain  Gain=M_n22
  Sum : Sum  Inputs=|+-
  Sum1 : Sum  Inputs=|+-
  Sum2 : Sum  Inputs=|++
  Torque_ref : Outport
  wires:
  Sum/1 -> Gain/1
  Position/1 -> Sum/2
  Position_cmd/1 -> Sum/1
  Sum1/1 -> Gain1/1
  Velocity_cmd/1 -> Sum1/1
  Velocity/1 -> Sum1/2
  Gain/1 -> Sum2/1
  Gain1/1 -> Sum2/2
  Sum2/1 -> Gain2/1
  Gain2/1 -> Torque_ref/1
